simulink library "ESTS"  (R2024b)
settings: Solver=VariableStepAuto  StartTime=0.0  StopTime=10.0  RelTol=1e-3
libraries: simulink x2, ESTS_FRIC x1, ESTS_LSM x1, ESTS_UOD x1, ESTS_VHSO x1, ESTS_VGMG x1, ESTS_VVSO x1
settings Model: Creator=blatak  LastModifiedBy=blatak
settings ModelReferenceCC: EnableRefExpFcnMdlSchedulingChecks=on
settings RTWCC: GPUComputeCapability=3.5

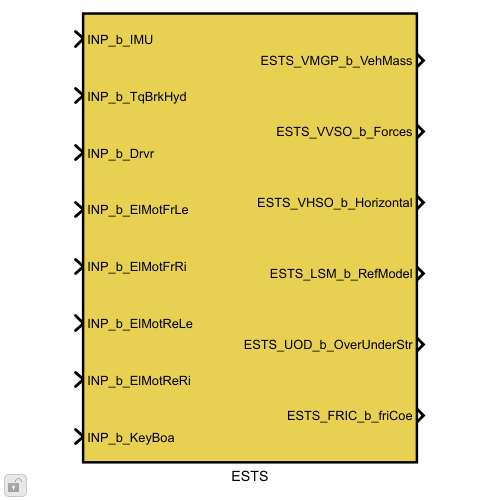
[thumbnail: Simulink's stored preview of the top-level diagram]
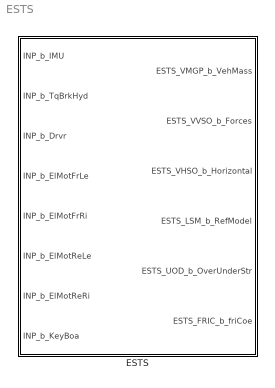
== system ESTS ==
  ESTS : Subsystem  TreatAsAtomicUnit=on

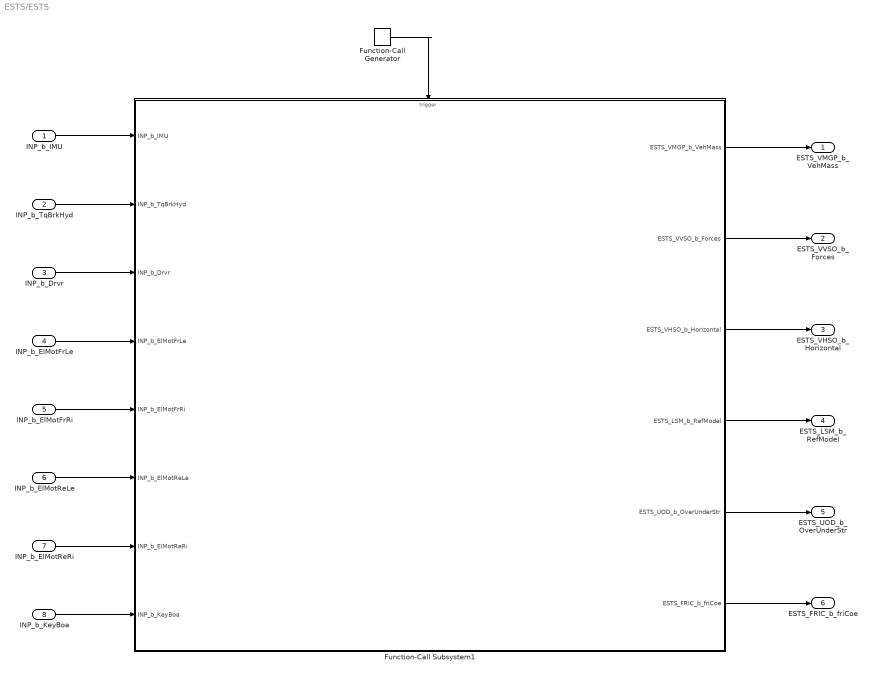
== system ESTS/ESTS ==
  INP_b_IMU : Inport
  INP_b_TqBrkHyd : Inport  Port=2
  INP_b_Drvr : Inport  Port=3
  INP_b_ElMotFrLe : Inport  Port=4
  INP_b_ElMotFrRi : Inport  Port=5
  INP_b_ElMotReLe : Inport  Port=6
  INP_b_ElMotReRi : Inport  Port=7
  INP_b_KeyBoa : Inport  Port=8
  Function-Call Generator : simulink/Ports & Subsystems/Function-Call Generator  sample_time=0.005  numberOfIterations=1  DisallowWideOutput=off
  Function-Call Subsystem1 : Subsystem  TreatAsAtomicUnit=on
  ESTS_VMGP_b_VehMass : Outport
  ESTS_VVSO_b_Forces : Outport  Port=2
  ESTS_VHSO_b_Horizontal : Outport  Port=3
  ESTS_LSM_b_RefModel : Outport  Port=4
  ESTS_UOD_b_OverUnderStr : Outport  Port=5
  ESTS_FRIC_b_friCoe : Outport  Port=6
  wires:
  INP_b_IMU/1 -> Function-Call Subsystem1/1(INP_b_IMU)
  INP_b_TqBrkHyd/1 -> Function-Call Subsystem1/2(INP_b_TqBrkHyd)
  INP_b_Drvr/1 -> Function-Call Subsystem1/3(INP_b_Drvr)
  INP_b_ElMotFrLe/1 -> Function-Call Subsystem1/4(INP_b_ElMotFrLe)
  INP_b_ElMotFrRi/1 -> Function-Call Subsystem1/5(INP_b_ElMotFrRi)
  INP_b_ElMotReLe/1 -> Function-Call Subsystem1/6(INP_b_ElMotReLe)
  INP_b_ElMotReRi/1 -> Function-Call Subsystem1/7(INP_b_ElMotReRi)
  Function-Call Generator/1 -> Function-Call Subsystem1/Trigger
  Function-Call Subsystem1/1(ESTS_VMGP_b_VehMass) -> ESTS_VMGP_b_VehMass/1
  Function-Call Subsystem1/2(ESTS_VVSO_b_Forces) -> ESTS_VVSO_b_Forces/1
  Function-Call Subsystem1/3(ESTS_VHSO_b_Horizontal) -> ESTS_VHSO_b_Horizontal/1
  Function-Call Subsystem1/4(ESTS_LSM_b_RefModel) -> ESTS_LSM_b_RefModel/1
  Function-Call Subsystem1/5(ESTS_UOD_b_OverUnderStr) -> ESTS_UOD_b_OverUnderStr/1
  INP_b_KeyBoa/1 -> Function-Call Subsystem1/8(INP_b_KeyBoa)
  Function-Call Subsystem1/6(ESTS_FRIC_b_friCoe) -> ESTS_FRIC_b_friCoe/1

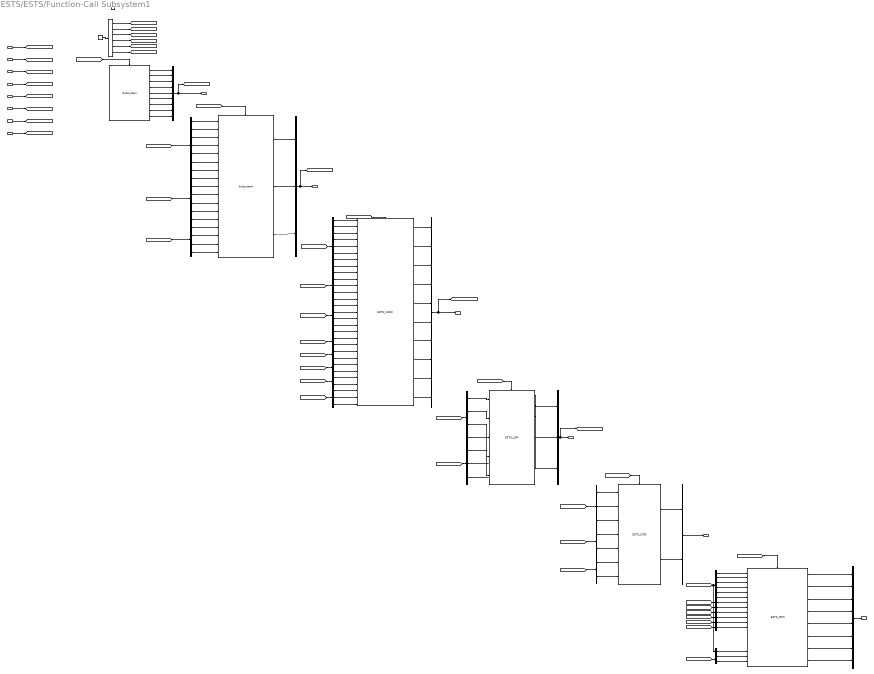
== system ESTS/ESTS/Function-Call Subsystem1 ==
  INP_b_IMU : Inport
  INP_b_TqBrkHyd : Inport  Port=2
  INP_b_Drvr : Inport  Port=3
  INP_b_ElMotFrLe : Inport  Port=4
  INP_b_ElMotFrRi : Inport  Port=5
  INP_b_ElMotReLe : Inport  Port=6
  INP_b_ElMotReRi : Inport  Port=7
  INP_b_KeyBoa : Inport  Port=8
  function : TriggerPort  TriggerType=function-call  VariantControl=(inherit)
  Bus Creator : BusCreator  Inputs=9  OutDataTypeStr=Bus: ESTS_VMGP_b_VehMass
      settings: InheritFromInputs=off
  Bus Creator1 : BusCreator  Inputs=3
  Bus Creator2 : BusCreator  Inputs=10  OutDataTypeStr=Bus: ESTS_VHSO_b_Horizontal
  Bus Creator3 : BusCreator  Inputs=8  OutDataTypeStr=Bus: ESTS_FRIC_b_friCoe
      settings: InheritFromInputs=off
  Bus Creator5 : BusCreator  Inputs=3
  Bus Creator6 : BusCreator  Inputs=2
  Bus Selector : BusSelector  OutputSignals=ESTS_VMGP_s_trackFr_m,ESTS_VMGP_s_trackRe_m,ESTS_VMGP_s_WhlBas_m,ESTS_VMGP_s_StatLoaFr_kg,ESTS_VMGP_s_StatLoaRe_kg,ESTS_VMGP_s_VehMas_kg,ESTS_VMGP_s_HeiCog_m
  Bus Selector1 : BusSelector  OutputSignals=INP_s_ALgtOfsCmp_mps2,INP_s_ALatOfsCmp_mps2,INP_s_AVertOfsCmp_mps2,INP_s_AngRatRollOfsCmp_radps,INP_s_AngRatPitchOfsCmp_radps,INP_s_AngRatYawOfsCmp_radps
  Bus Selector10 : BusSelector  OutputSignals=INP_EMFL_s_SpdMotFrLe_1pmin,INP_EMFL_s_TqMotFrLe_Nm
  Bus Selector11 : BusSelector  OutputSignals=INP_EMFR_s_SpdMotFrRi_1pmin,INP_EMFR_s_TqMotFrRi_Nm
  Bus Selector12 : BusSelector  OutputSignals=INP_EMRL_s_SpdMotReLe_1pmin,INP_EMRL_s_TqMotReLe_Nm
  Bus Selector13 : BusSelector  OutputSignals=INP_DRVR_s_AngStFrLe_rad,INP_DRVR_s_AngStFrRi_rad,INP_DRVR_s_AngStFr_rad
  Bus Selector14 : BusSelector  OutputSignals=INP_s_AngRatYawOfsCmp_radps,INP_s_ALatOfsCmp_mps2
  Bus Selector15 : BusSelector  OutputSignals=INP_EMRR_s_SpdMotReRi_1pmin,INP_EMRR_s_TqMotReRi_Nm
  Bus Selector16 : BusSelector  OutputSignals=ESTS_HVSO_s_VLatCog_mps,ESTS_HVSO_s_VLgtCog_mps,ESTS_HVSO_s1_FLatXxYy_N,ESTS_HVSO_s1_FLgtXxYy_N,ESTS_HVSO_s1_SlipWhl_p1,ESTS_HVSO_s_SlipAngCog_deg
  Bus Selector17 : BusSelector  OutputSignals=INP_KEY_s_ModFric_na
  Bus Selector18 : BusSelector  OutputSignals=ESTS_VVSO_s1_FVertXxYy_N
  Bus Selector19 : BusSelector  OutputSignals=INP_s_ALatOfsCmp_mps2,INP_s_ALgtOfsCmp_mps2
  Bus Selector2 : BusSelector  OutputSignals=ESTS_VMGP_s_trackFr_m,ESTS_VMGP_s_trackRe_m,ESTS_VMGP_s_WhlBas_m,ESTS_VMGP_s_StatLoaFr_kg,ESTS_VMGP_s_StatLoaRe_kg,ESTS_VMGP_s_VehMas_kg,ESTS_VMGP_s_HeiCog_m,ESTS_VMGP_s_DistCogAxlFr_m,ESTS_VMGP_s_DistCogAxlRe_m
  Bus Selector20 : BusSelector  OutputSignals=INP_EMFL_s_TqMotFrLe_Nm
  Bus Selector21 : BusSelector  OutputSignals=INP_EMFR_s_TqMotFrRi_Nm
  Bus Selector22 : BusSelector  OutputSignals=INP_EMRL_s_TqMotReLe_Nm
  Bus Selector23 : BusSelector  OutputSignals=INP_EMRR_s_TqMotReRi_Nm
  Bus Selector24 : BusSelector  OutputSignals=ESTS_HVSO_s_SpdRefVeh_mps
  Bus Selector3 : BusSelector  OutputSignals=ESTS_VVSO_s1_FVertXxYy_N,ESTS_VVSO_PitchAngle_rad,ESTS_VVSO_RollAngle_rad
  Bus Selector4 : BusSelector  OutputSignals=INP_s_ALgtOfsCmp_mps2,INP_s_ALatOfsCmp_mps2,INP_s_AVertOfsCmp_mps2,INP_s_AngRatRollOfsCmp_radps,INP_s_AngRatPitchOfsCmp_radps,INP_s_AngRatYawOfsCmp_radps
  Bus Selector5 : BusSelector  OutputSignals=ESTS_HVSO_s_SpdRefVeh_mps,ESTS_HVSO_s_VLgtCog_mps,ESTS_HVSO_s_SlipAngVelRe_radps
  Bus Selector6 : BusSelector  OutputSignals=INP_DRVR_s_AngStWhl_rad,INP_DRVR_s_PosThr_p100,INP_DRVR_s_RegGear_na,INP_DRVR_s_RegDrvSplit_na
  Bus Selector7 : BusSelector  OutputSignals=ESTS_LSM_s_AngRatYawRef_radps,ESTS_LSM_s_SlipAngRef_rad,ESTS_LSM_s_RearSlipAngleVel_radps
  Bus Selector8 : BusSelector  OutputSignals=ESTS_HVSO_s_SpdRefVeh_mps,ESTS_HVSO_s_SlipAngVelRe_radps
  Bus Selector9 : BusSelector  OutputSignals=INP_DRVR_s_AngStWhl_rad,INP_DRVR_s_PosThr_p100,INP_DRVR_s_RegGear_na,INP_DRVR_s_RegDrvSplit_na
  ESTS_FRIC : ESTS_FRIC/ESTS_FRIC  SystemSampleTime=-1  VariantActivationTime=update diagram  AllowFlexibleInterface=on  Latency=0  AutoFrameSizeCalculation=off
  ESTS_LSM : ESTS_LSM/ESTS_LSM  SystemSampleTime=-1  VariantActivationTime=update diagram  AllowFlexibleInterface=on  Latency=0  AutoFrameSizeCalculation=off
  ESTS_UOD1 : ESTS_UOD/ESTS_UOD  SystemSampleTime=-1  VariantActivationTime=update diagram  AllowFlexibleInterface=on  Latency=0  AutoFrameSizeCalculation=off
  ESTS_VHSO : ESTS_VHSO/ESTS_VHSO  SystemSampleTime=-1  VariantActivationTime=update diagram  AllowFlexibleInterface=on  Latency=0  AutoFrameSizeCalculation=off
  Function-Call Generator : simulink/Ports & Subsystems/Function-Call Generator  sample_time=-1  numberOfIterations=1  DisallowWideOutput=off
  Function-Call Split : FunctionCallSplit  IconShape=distinctive  NumOutputPorts=6  OutputPortLayout=default
  Subsystem1 : ESTS_VGMG/Subsystem  SystemSampleTime=-1  VariantActivationTime=update diagram  AllowFlexibleInterface=on  Latency=0  AutoFrameSizeCalculation=off
  Subsystem2 : ESTS_VVSO/Subsystem  SystemSampleTime=-1  VariantActivationTime=update diagram  AllowFlexibleInterface=on  Latency=0  AutoFrameSizeCalculation=off
  ESTS_VMGP_b_VehMass : Outport
  ESTS_VVSO_b_Forces : Outport  Port=2
  ESTS_VHSO_b_Horizontal : Outport  Port=3
  ESTS_LSM_b_RefModel : Outport  Port=4
  ESTS_UOD_b_OverUnderStr : Outport  Port=5
  ESTS_FRIC_b_friCoe : Outport  Port=6
  wires:
  Subsystem1/6 -> Bus Creator/6  "ESTS_VMGP_s_VehMas_kg"
  Bus Creator/1 -> ESTS_VMGP_b_VehMass/1, [ESTS_VMGP_b_VehMass]
  Bus Selector/5 -> Subsystem2/5  "<ESTS_VMGP_s_StatLoaRe_kg>"
  Subsystem1/1 -> Bus Creator/1  "ESTS_VMGP_s_trackFr_m"
  Subsystem1/4 -> Bus Creator/4  "ESTS_VMGP_s_StatLoaFr_kg"
  Bus Selector/6 -> Subsystem2/6  "<ESTS_VMGP_s_VehMas_kg>"
  Bus Selector1/6 -> Subsystem2/13  "<INP_s_AngRatYawOfsCmp_radps>"
  Bus Selector/4 -> Subsystem2/4  "<ESTS_VMGP_s_StatLoaFr_kg>"
  Bus Selector/1 -> Subsystem2/1  "<ESTS_VMGP_s_trackFr_m>"
  INP_b_TqBrkHyd/1 -> [INP_b_TqBrkHyd]
  Subsystem1/3 -> Bus Creator/3  "ESTS_VMGP_s_WhlBas_m"
  Bus Creator1/1 -> [ESTS_VVSO_b_Forces], ESTS_VVSO_b_Forces/1
  INP_b_IMU/1 -> [INP_b_IMU]
  Subsystem2/2 -> Bus Creator1/2  "ESTS_VVSO_PitchAngle_rad"
  Bus Selector1/5 -> Subsystem2/12  "<INP_s_AngRatPitchOfsCmp_radps>"
  INP_b_Drvr/1 -> [INP_b_Drvr]
  Bus Selector1/1 -> Subsystem2/8  "<INP_s_ALgtOfsCmp_mps2>"
  Bus Selector1/4 -> Subsystem2/11  "<INP_s_AngRatRollOfsCmp_radps>"
  Bus Selector/3 -> Subsystem2/3  "<ESTS_VMGP_s_WhlBas_m>"
  Subsystem2/1 -> Bus Creator1/1  "ESTS_VVSO_s1_FVertXxYy_N"
  Bus Selector/2 -> Subsystem2/2  "<ESTS_VMGP_s_trackRe_m>"
  [ESTS_VMGP_b_VehMass] -> Bus Selector/1
  INP_b_ElMotReRi/1 -> [INP_b_ElMotReRi]
  INP_b_ElMotReLe/1 -> [INP_b_ElMotReLe]
  Subsystem1/2 -> Bus Creator/2  "ESTS_VMGP_s_trackRe_m"
  Subsystem1/7 -> Bus Creator/7  "ESTS_VMGP_s_HeiCog_m"
  Subsystem1/5 -> Bus Creator/5  "ESTS_VMGP_s_StatLoaRe_kg"
  INP_b_ElMotFrRi/1 -> [INP_b_ElMotFrRi]
  Bus Selector/7 -> Subsystem2/7  "<ESTS_VMGP_s_HeiCog_m>"
  Bus Selector1/3 -> Subsystem2/10  "<INP_s_AVertOfsCmp_mps2>"
  Bus Selector1/2 -> Subsystem2/9  "<INP_s_ALatOfsCmp_mps2>"
  INP_b_ElMotFrLe/1 -> [INP_b_ElMotFrLe]
  Subsystem2/3 -> Bus Creator1/3  "ESTS_VVSO_RollAngle_rad"
  Function-Call Generator/1 -> Function-Call Split/1
  Function-Call Split/1 -> [fc_ESTS_VMGP]
  [fc_ESTS_VMGP] -> Subsystem1/Trigger
  [fc_ESTS_VVSO] -> Subsystem2/Trigger
  Function-Call Split/2 -> [fc_ESTS_VVSO]
  [fc_ESTS_VHSO] -> ESTS_VHSO/Trigger
  Function-Call Split/3 -> [fc_ESTS_VHSO]
  Function-Call Split/4 -> [fc_ESTS_LSM]
  [fc_ESTS_LSM] -> ESTS_LSM/Trigger
  Function-Call Split/5 -> [fc_ESTS_UOD]
  [fc_ESTS_UOD] -> ESTS_UOD1/Trigger
  Bus Selector2/2 -> ESTS_VHSO/2  "<ESTS_VMGP_s_trackRe_m>"
  [ESTS_VMGP_b_VehMass] -> Bus Selector2/1
  ESTS_VHSO/1 -> Bus Creator2/1  "ESTS_HVSO_s_SpdRefVeh_mps"
  ESTS_VHSO/2 -> Bus Creator2/2  "ESTS_HVSO_s_VLatCog_mps"
  ESTS_VHSO/3 -> Bus Creator2/3  "ESTS_HVSO_s_VLgtCog_mps"
  ESTS_VHSO/4 -> Bus Creator2/4  "ESTS_HVSO_s1_FLatXxYy_N"
  ESTS_VHSO/5 -> Bus Creator2/5  "ESTS_HVSO_s1_FLgtXxYy_N"
  ESTS_VHSO/6 -> Bus Creator2/6  "ESTS_HVSO_s1_SlipWhl_p1"
  ESTS_VHSO/7 -> Bus Creator2/7  "ESTS_HVSO_s_SlipAngCog_deg"
  ESTS_VHSO/8 -> Bus Creator2/8  "ESTS_HVSO_s_AngRoadBnk_deg"
  ESTS_VHSO/9 -> Bus Creator2/9  "ESTS_HVSO_s_AngRoadSlop_deg"
  ESTS_VHSO/10 -> Bus Creator2/10  "ESTS_HVSO_s_SlipAngVelRe_radps"
  Bus Creator2/1 -> [ESTS_VHSO_b_Horizontal], ESTS_VHSO_b_Horizontal/1
  [ESTS_VVSO_b_Forces] -> Bus Selector3/1
  [INP_b_IMU] -> Bus Selector4/1
  Bus Selector3/3 -> ESTS_VHSO/12  "<ESTS_VVSO_RollAngle_rad>"
  Bus Selector3/2 -> ESTS_VHSO/11  "<ESTS_VVSO_PitchAngle_rad>"
  Bus Selector3/1 -> ESTS_VHSO/10  "<ESTS_VVSO_s1_FVertXxYy_N>"
  Bus Selector2/1 -> ESTS_VHSO/1  "<ESTS_VMGP_s_trackFr_m>"
  Bus Selector2/3 -> ESTS_VHSO/3  "<ESTS_VMGP_s_WhlBas_m>"
  Bus Selector2/4 -> ESTS_VHSO/4  "<ESTS_VMGP_s_StatLoaFr_kg>"
  Bus Selector2/5 -> ESTS_VHSO/5  "<ESTS_VMGP_s_StatLoaRe_kg>"
  Bus Selector2/6 -> ESTS_VHSO/6  "<ESTS_VMGP_s_VehMas_kg>"
  Bus Selector2/7 -> ESTS_VHSO/7  "<ESTS_VMGP_s_HeiCog_m>"
  Bus Selector4/1 -> ESTS_VHSO/13  "<INP_s_ALgtOfsCmp_mps2>"
  Bus Selector4/2 -> ESTS_VHSO/14  "<INP_s_ALatOfsCmp_mps2>"
  Bus Selector4/3 -> ESTS_VHSO/15  "<INP_s_AVertOfsCmp_mps2>"
  Bus Selector4/4 -> ESTS_VHSO/16  "<INP_s_AngRatRollOfsCmp_radps>"
  Bus Selector4/5 -> ESTS_VHSO/17  "<INP_s_AngRatPitchOfsCmp_radps>"
  Bus Selector4/6 -> ESTS_VHSO/18  "<INP_s_AngRatYawOfsCmp_radps>"
  [ESTS_VHSO_b_Horizontal] -> Bus Selector5/1
  [INP_b_Drvr] -> Bus Selector6/1
  Bus Selector6/1 -> ESTS_LSM/1  "<INP_DRVR_s_AngStWhl_rad>"
  Bus Selector6/2 -> ESTS_LSM/2  "<INP_DRVR_s_PosThr_p100>"
  ESTS_LSM/1 -> Bus Creator5/1  "ESTS_LSM_s_AngRatYawRef_radps"
  ESTS_LSM/2 -> Bus Creator5/2  "ESTS_LSM_s_SlipAngRef_rad"
  Bus Creator5/1 -> ESTS_LSM_b_RefModel/1, [ESTS_LSM_b_RefModel]
  ESTS_LSM/3 -> Bus Creator5/3  "ESTS_LSM_s_RearSlipAngleVel_radps"
  [ESTS_LSM_b_RefModel] -> Bus Selector7/1
  [ESTS_VHSO_b_Horizontal] -> Bus Selector8/1
  Bus Selector7/2 -> ESTS_UOD1/2  "<ESTS_LSM_s_SlipAngRef_rad>"
  Bus Selector7/3 -> ESTS_UOD1/3  "<ESTS_LSM_s_RearSlipAngleVel_radps>"
  Bus Selector7/1 -> ESTS_UOD1/1  "<ESTS_LSM_s_AngRatYawRef_radps>"
  Bus Selector8/1 -> ESTS_UOD1/4  "<ESTS_HVSO_s_SpdRefVeh_mps>"
  Bus Selector8/2 -> ESTS_UOD1/5  "<ESTS_HVSO_s_SlipAngVelRe_radps>"
  ESTS_UOD1/2 -> Bus Creator6/2  "ESTS_UOD_s_Overstr_p1"
  ESTS_UOD1/1 -> Bus Creator6/1  "ESTS_UOD_s_Undrstr_p1"
  Bus Creator6/1 -> ESTS_UOD_b_OverUnderStr/1
  Bus Selector9/1 -> Subsystem2/14  "<INP_DRVR_s_AngStWhl_rad>"
  Bus Selector9/2 -> Subsystem2/15  "<INP_DRVR_s_PosThr_p100>"
  [INP_b_Drvr] -> Bus Selector9/1
  [INP_b_IMU] -> Bus Selector1/1
  Bus Selector9/3 -> Subsystem2/16  "<INP_DRVR_s_RegGear_na>"
  Bus Selector9/4 -> Subsystem2/17  "<INP_DRVR_s_RegDrvSplit_na>"
  Bus Selector6/3 -> ESTS_LSM/3  "<INP_DRVR_s_RegGear_na>"
  Bus Selector6/4 -> ESTS_LSM/4  "<INP_DRVR_s_RegDrvSplit_na>"
  Bus Selector5/1 -> ESTS_LSM/5  "<ESTS_HVSO_s_SpdRefVeh_mps>"
  Bus Selector5/2 -> ?  "<ESTS_HVSO_s_VLgtCog_mps>"
  Bus Selector5/3 -> ?  "<ESTS_HVSO_s_SlipAngVelRe_radps>"
  [INP_b_ElMotFrLe] -> Bus Selector10/1
  Bus Selector10/1 -> ESTS_VHSO/19  "<INP_EMFL_s_SpdMotFrLe_1pmin>"
  Bus Selector10/2 -> ESTS_VHSO/20  "<INP_EMFL_s_TqMotFrLe_Nm>"
  Bus Selector11/1 -> ESTS_VHSO/21  "<INP_EMFR_s_SpdMotFrRi_1pmin>"
  Bus Selector11/2 -> ESTS_VHSO/22  "<INP_EMFR_s_TqMotFrRi_Nm>"
  Bus Selector12/1 -> ESTS_VHSO/23  "<INP_EMRL_s_SpdMotReLe_1pmin>"
  Bus Selector12/2 -> ESTS_VHSO/24  "<INP_EMRL_s_TqMotReLe_Nm>"
  Bus Selector15/1 -> ESTS_VHSO/25  "<INP_EMRR_s_SpdMotReRi_1pmin>"
  Bus Selector15/2 -> ESTS_VHSO/26  "<INP_EMRR_s_TqMotReRi_Nm>"
  Subsystem1/8 -> Bus Creator/8  "ESTS_VMGP_s_DistCogAxlFr_m"
  Subsystem1/9 -> Bus Creator/9  "ESTS_VMGP_s_DistCogAxlRe_m"
  Bus Selector2/8 -> ESTS_VHSO/8  "<ESTS_VMGP_s_DistCogAxlFr_m>"
  Bus Selector2/9 -> ESTS_VHSO/9  "<ESTS_VMGP_s_DistCogAxlRe_m>"
  [INP_b_Drvr] -> Bus Selector13/1
  Bus Selector13/1 -> ESTS_VHSO/27  "<INP_DRVR_s_AngStFrLe_rad>"
  Bus Selector13/2 -> ESTS_VHSO/28  "<INP_DRVR_s_AngStFrRi_rad>"
  Bus Selector13/3 -> ESTS_VHSO/29  "<INP_DRVR_s_AngStFr_rad>"
  [INP_b_IMU] -> Bus Selector14/1
  Bus Selector14/1 -> ESTS_UOD1/6  "<INP_s_AngRatYawOfsCmp_radps>"
  Bus Selector14/2 -> ESTS_UOD1/7  "<INP_s_ALatOfsCmp_mps2>"
  INP_b_KeyBoa/1 -> [INP_b_KeyBoa]
  [INP_b_ElMotFrRi] -> Bus Selector11/1
  [INP_b_ElMotReRi] -> Bus Selector15/1
  [INP_b_ElMotReLe] -> Bus Selector12/1
  Function-Call Split/6 -> [fc_ESTS_FRIC]
  [fc_ESTS_FRIC] -> ESTS_FRIC/Trigger
  [ESTS_VHSO_b_Horizontal] -> Bus Selector24/1, Bus Selector16/1
  [INP_b_KeyBoa] -> Bus Selector17/1
  Bus Selector16/1 -> ESTS_FRIC/1  "<ESTS_HVSO_s_VLatCog_mps>"
  Bus Selector16/2 -> ESTS_FRIC/2  "<ESTS_HVSO_s_VLgtCog_mps>"
  Bus Selector16/3 -> ESTS_FRIC/3  "<ESTS_HVSO_s1_FLatXxYy_N>"
  Bus Selector16/4 -> ESTS_FRIC/4  "<ESTS_HVSO_s1_FLgtXxYy_N>"
  Bus Selector16/5 -> ESTS_FRIC/5  "<ESTS_HVSO_s1_SlipWhl_p1>"
  Bus Selector16/6 -> ESTS_FRIC/6  "<ESTS_HVSO_s_SlipAngCog_deg>"
  Bus Selector17/1 -> ESTS_FRIC/8  "<INP_KEY_s_ModFric_na>"
  [ESTS_VVSO_b_Forces] -> Bus Selector18/1
  Bus Selector18/1 -> ESTS_FRIC/7  "<ESTS_VVSO_s1_FVertXxYy_N>"
  Bus Creator3/1 -> ESTS_FRIC_b_friCoe/1
  ESTS_FRIC/1 -> Bus Creator3/1  "ESTS_FRIC_SLIP_s_FriCoe_na"
  ESTS_FRIC/2 -> Bus Creator3/2  "ESTS_FRIC_SLIP_s_FriCoeActFrLe_na"
  ESTS_FRIC/3 -> Bus Creator3/3  "ESTS_FRIC_SLIP_s_FriCoeActFrRi_na"
  ESTS_FRIC/4 -> Bus Creator3/4  "ESTS_FRIC_SLIP_s_FriCoeActReLe_na"
  ESTS_FRIC/5 -> Bus Creator3/5  "ESTS_FRIC_SLIP_s_FriCoeActReRi_na"
  ESTS_FRIC/6 -> Bus Creator3/6  "ESTS_FRIC_SLIP_s_FriCoeAvg_na"
  ESTS_FRIC/7 -> Bus Creator3/7  "ESTS_FRIC_SLIP_s_FriCoeAvgMovAvg_na"
  ESTS_FRIC/8 -> Bus Creator3/8  "ESTS_FRIC_HILO_STATE_s_FlgLowMue_na"
  Bus Selector19/1 -> ESTS_FRIC/18  "<INP_s_ALatOfsCmp_mps2>"
  Bus Selector19/2 -> ESTS_FRIC/19  "<INP_s_ALgtOfsCmp_mps2>"
  [INP_b_IMU] -> Bus Selector19/1
  Bus Selector20/1 -> ESTS_FRIC/9  "<INP_EMFL_s_TqMotFrLe_Nm>"
  Bus Selector21/1 -> ESTS_FRIC/10  "<INP_EMFR_s_TqMotFrRi_Nm>"
  [INP_b_ElMotFrRi] -> Bus Selector21/1
  Bus Selector22/1 -> ESTS_FRIC/11  "<INP_EMRL_s_TqMotReLe_Nm>"
  Bus Selector23/1 -> ESTS_FRIC/12  "<INP_EMRR_s_TqMotReRi_Nm>"
  [INP_b_ElMotReRi] -> Bus Selector23/1
  [INP_b_ElMotFrLe] -> Bus Selector20/1
  [INP_b_ElMotReLe] -> Bus Selector22/1
  Bus Selector24/1 -> ESTS_FRIC/17  "<ESTS_HVSO_s_SpdRefVeh_mps>"
